simulink model "ip02_quick_start"  (Simulink 7.8)
settings: Solver=ode1  StartTime=0.0  StopTime=inf  FixedStep=0.002  RelTol=1e-3
PostLoadFcn:
  | qc_set_target_type(getConfigSet(bdroot, 'QUARC Default Target Configuration'));
undefined symbols (not defined in the file): HIL
libraries: quarc_library x3, simulink x1, simulink_extras x1
settings Model: Creator=pmartin  LastModifiedBy=pmartin  SimulationMode=external  ExtModeTrigDuration=5000
settings SolverCC: PositivePriorityOrder=on
settings OptimizationCC: InitFltsAndDblsToZero=on
settings DebuggingCC: SaveWithParameterizedLinksMsg=none  MultiTaskDSMMsg=warning  MultiTaskCondExecSysMsg=none  FcnCallInpInsideContextMsg=Use local settings  StrictBusMsg=None
settings RTWCC: SystemTargetFile=quarc_windows.tlc  TemplateMakefile=quarc_default_tmf  Description=QUARC Win32 Target  ProcessScript=quarc_windows_make_rtw_hook
settings STFCustomTargetCC: TargetPreCompLibLocation=C:\PROGRA~2\QUARC\lib\2012b\windows\release  CombineOutputUpdateFcns=on  SystemTargetFile=quarc_windows.tlc
settings GRTTargetCC: TargetPreCompLibLocation=C:\PROGRA~2\QUARC\lib\2012b\windows\release  ParMdlRefBuildCompliant=off  CompOptLevelCompliant=off  ConcurrentExecutionCompliant=off  CombineOutputUpdateFcns=on  MatFileLogging=off  ExtMode=on  ExtModeMexFile=quarc_comm

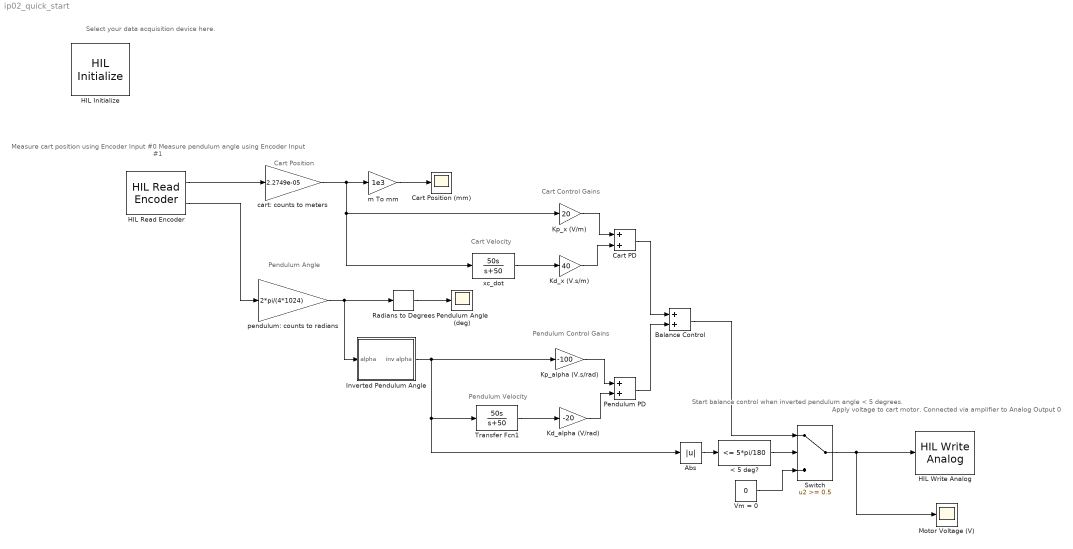
== system ip02_quick_start ==
  note: Measure cart position using Encoder Input #0
      | Measure pendulum angle using Encoder Input #1
  note: Cart Control Gains
  note: Pendulum Angle
  note: Cart Velocity
  note: Start balance control
      |  when inverted pendulum
      | angle < 5 degrees.
  note: Cart Position
  note: Pendulum Velocity
  note: Pendulum Control Gains
  note: Apply voltage to cart motor.
      | Connected via amplifier to Analog Output 0
  note: Select your data acquisition device here.
  < 5 deg? : simulink/Logic and Bit Operations/Compare To Constant  relop=<=  const=5*pi/180  OutDataTypeStr=boolean
  Abs : Abs
  Balance Control : Sum
  Cart PD : Sum
  Cart Position (mm) : Scope
      settings: TickLabels=on  TimeRange=10  YMin=-80  YMax=70  SaveName=data_xc
  HIL Initialize : quarc_library/Data Acquisition/Generic/Configuration/HIL Initialize  object_name=HIL-1  board_type=q2_usb  board_number=0  board_options=d0=digital;d1=digital;led=auto;update_rate=normal  exclusive=off  active=off  hardware_clocks=[0:2]  clock_modes=[]  initial_clock_frequencies=[]  set_clock_params_at_start=off  set_clock_params_at_switch_in=off  set_clock_frequencies_at_start=off  set_clock_frequencies_at_switch_in=off  analog_input_channels=[0:1]  analog_input_maximums=10  analog_input_minimums=-10  set_analog_input_params_at_start=on  set_analog_input_params_at_switch_in=off  analog_output_channels=[0:1]  analog_output_maximums=10  analog_output_minimums=-10  initial_analog_outputs=[0]  final_analog_outputs=[0]  watchdog_analog_outputs=0  set_analog_output_params_at_start=on  set_analog_output_params_at_switch_in=off  set_analog_outputs_at_start=on  set_analog_outputs_at_switch_in=off  set_analog_outputs_at_terminate=on  set_analog_outputs_at_switch_out=off  set_analog_outputs_on_watchdog=off  digital_input_channels=[]  digital_output_channels=[0:7]  digital_output_configuration=[]  initial_digital_outputs=[0]  final_digital_outputs=[0]  watchdog_digital_outputs=[0]  set_digital_output_params_at_start=off  set_digital_output_params_at_switch_in=off  set_digital_outputs_at_start=on  set_digital_outputs_at_switch_in=off  set_digital_outputs_at_terminate=on  set_digital_outputs_at_switch_out=off  set_digital_outputs_on_watchdog=off  encoder_channels=[0:1]  quadrature=[4]  encoder_filter_frequency=[]  initial_encoder_counts=[0]  set_encoder_params_at_start=on  set_encoder_params_at_switch_in=off  set_encoder_counts_at_start=on  set_encoder_counts_at_switch_in=off  pwm_channels=[]  pwm_modes=[0]  pwm_frequency=1/0.020  pwm_configuration=[]  pwm_alignment=[]  pwm_polarity=[]  pwm_leading_deadband=[]  pwm_trailing_deadband=[]  initial_pwm_outputs=[0]  final_pwm_outputs=[0]  watchdog_pwm_outputs=[0]  set_pwm_params_at_start=on  set_pwm_params_at_switch_in=off  set_pwm_outputs_at_start=on  set_pwm_outputs_at_switch_in=off  set_pwm_outputs_at_terminate=on  set_pwm_outputs_at_switch_out=off  set_pwm_outputs_on_watchdog=off  other_output_channels=[]  initial_other_outputs=[]  final_other_outputs=[]  watchdog_other_outputs=[]  set_other_outputs_at_start=off  set_other_outputs_at_switch_in=off  set_other_outputs_at_terminate=off  set_other_outputs_at_switch_out=off  set_other_outputs_on_watchdog=off
  HIL Read Encoder : quarc_library/Data Acquisition/Generic/Immediate I//O/HIL Read Encoder  object_name=HIL-1  channels=[0:1]  sample_time=qc_get_step_size  active=on  vector_output=off  data_type_mode=Inherit via back propagation  data_type=double
  HIL Write Analog : quarc_library/Data Acquisition/Generic/Immediate I//O/HIL Write Analog  object_name=HIL-1  channels=0  sample_time=-1  active=off  vector_input=off
  Inverted Pendulum Angle : Subsystem
  Kd_alpha (V/rad) : Gain  Gain=-20
  Kd_x (V.s/m) : Gain  Gain=40
  Kp_alpha (V.s/rad) : Gain  Gain=-100
  Kp_x (V/m) : Gain  Gain=20
  Motor Voltage (V) : Scope
  Pendulum Angle (deg) : Scope
      settings: TickLabels=on  TimeRange=10  YMin=-180  YMax=10  SaveName=data_alpha
  Pendulum PD : Sum
  Radians to Degrees : simulink_extras/Transformations/Radians to Degrees
  Switch : Switch  Threshold=0.5
  Transfer Fcn1 : TransferFcn  Numerator=[50 0]  Denominator=[1 50]
  Vm = 0 : Constant  Value=0
  cart: counts to meters : Gain  Gain=2.2749e-05  SaturateOnIntegerOverflow=on  OutDataTypeStr=Inherit: Same as input  ParamDataTypeStr=Inherit: Same as input
  m To mm : Gain  Gain=1e3  SaturateOnIntegerOverflow=on  OutDataTypeStr=Inherit: Same as input  ParamDataTypeStr=Inherit: Same as input
  pendulum: counts to radians : Gain  Gain=2*pi/(4*1024)  SaturateOnIntegerOverflow=on  OutDataTypeStr=Inherit: Same as input  ParamDataTypeStr=Inherit: Same as input
  xc_dot : TransferFcn  Numerator=[50 0]  Denominator=[1 50]
  wires:
  m To mm/1 -> Cart Position (mm)/1
  Radians to Degrees/1 -> Pendulum Angle (deg)/1
  HIL Read Encoder/1 -> cart: counts to meters/1
  HIL Read Encoder/2 -> pendulum: counts to radians/1
  Vm = 0/1 -> Switch/3
  cart: counts to meters/1 -> Kp_x (V/m)/1, xc_dot/1, m To mm/1
  pendulum: counts to radians/1 -> Inverted Pendulum Angle/1(alpha), Radians to Degrees/1
  Abs/1 -> < 5 deg?/1
  < 5 deg?/1 -> Switch/2
  Switch/1 -> Motor Voltage (V)/1, HIL Write Analog/1
  Balance Control/1 -> Switch/1
  xc_dot/1 -> Kd_x (V.s/m)/1
  Transfer Fcn1/1 -> Kd_alpha (V/rad)/1
  Kd_x (V.s/m)/1 -> Cart PD/2
  Kp_x (V/m)/1 -> Cart PD/1
  Kd_alpha (V/rad)/1 -> Pendulum PD/2
  Kp_alpha (V.s/rad)/1 -> Pendulum PD/1
  Cart PD/1 -> Balance Control/1
  Pendulum PD/1 -> Balance Control/2
  Inverted Pendulum Angle/1(inv alpha) -> Abs/1, Transfer Fcn1/1, Kp_alpha (V.s/rad)/1

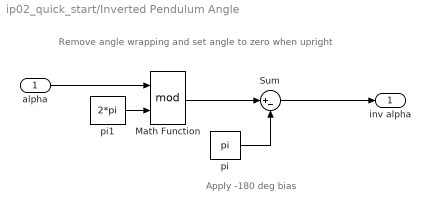
== system ip02_quick_start/Inverted Pendulum Angle ==
  note: Apply -180 deg bias
  note: Remove angle wrapping and
      | set angle to zero when upright
  alpha : Inport
  Math Function : Math  Operator=mod  SaturateOnIntegerOverflow=on
  Sum : Sum  Inputs=|+-  SaturateOnIntegerOverflow=on  InputSameDT=on  OutDataTypeStr=Inherit: Same as first input
  pi : Constant  Value=pi
  pi1 : Constant  Value=2*pi
  inv alpha : Outport  InitialOutput=0
  wires:
  alpha/1 -> Math Function/1
  pi/1 -> Sum/2
  pi1/1 -> Math Function/2
  Sum/1 -> inv alpha/1
  Math Function/1 -> Sum/1
